simulink model "dbt_ut"  (Simulink 8.1)
settings: Solver=FixedStepDiscrete  StartTime=0.0  StopTime=Inf  FixedStep=0.005  RelTol=1e-3
PostLoadFcn:
  | , if any(exist('dsrtsu_mdlpostloadfcn', 'file') == [2, 3, 6]), try dsrtsu_mdlpostloadfcn('Execute', bdroot); catch fprintf('Error in PostLoadFcn (dsrtsu_mdlpostloadfcn) for model "%s":\n %s\n', bdroot, lasterr); end, end,
libraries: siltestlib x6, dbt x1
settings Model: DSRTSU_INTERNAL_RTI_VER=450  DSRTSU_INTERNAL_RTI_TYPE=rti1401  RTICANMMDATA=struct('GeneralSetupData',struct('modelroot','D:\ELN150201_TAIWAN\trunk\AdasDragon\software\sw_development\arch\app\acc','generalsettings',struct('filesettings',struct('destfolder',struct('Name','RTICANMM_FILES','Check',1),'buildfolder',struct('Name','.','Check',1),'AbsDestfolder',struct('Name','D:\ELN150201_TAIWAN\trunk\AdasDragon\software\sw_development\arch\app\acc\RTICANMM_FILES'),'AbsBuildfolder',struct('Name','D:\ELN150201_TAIWAN\trunk\AdasDragon\software\sw_development\arch\app\acc'))),'options',struct('addpaths',1,'rmpaths',1,'addtrcexclusion',logical(1),'cannavigator',struct('checkmonitoring',0),'show_usrtrc',0,'use_usrtrc',0),'advanced',struct('options',[1 1 1 1 1 1 1 1 1 1 1 1 1 1 1 1 1 1 1 1 1 1 1 1 1 1 1 1 1 1 1 1 1 1 1 1 1 1 1 1 1 1 1 1 1 1 1 1 1 1 1 1 1 1 1 1 1 1 1 1 1 1 1 1 1 1 1 1 1 1 1 1 1 1 1 1 1 1 1 1 1 1 1 1 1 1 1 1 1 1 1 1 1 1 1 1 1 1 1 1]),'MPSetup',{{}},'modelname','dbt_ut','block','dbt_ut'))  DSRTSU_INTERNAL_RTIFPGA=40  Creator=AT015555  LastModifiedBy=AT015555  BufferReuse=off
settings DataIOCC: SignalLoggingSaveFormat=Dataset
settings OptimizationCC: BlockReduction=off  OptimizeBlockIOStorage=off  BufferReuse=off  ExpressionFolding=off  ExpressionDepthLimit=128  LocalBlockOutputs=off
settings DebuggingCC: FcnCallInpInsideContextMsg=EnableAllAsError
settings HardwareCC: ProdIntDivRoundTo=Zero  ProdEndianess=BigEndian  ProdHWDeviceType=Generic->Custom  TargetIntDivRoundTo=Zero  TargetEndianess=BigEndian  TargetHWDeviceType=Generic->Custom
settings RTWCC: SystemTargetFile=rti1401.tlc  MakeCommand=make_rti  TemplateMakefile=rti1401.tmf  Description=dSPACE DS1401 Hardware Platform  ProcessScript=rti1401_make_rtw_hook
settings STFCustomTargetCC: CodeReplacementLibrary=ANSI_C  ParMdlRefBuildCompliant=on  GeneratePreprocessorConditionals=Disable all  MatFileLogging=on  SystemTargetFile=rti1401.tlc
settings GRTTargetCC: CompOptLevelCompliant=off  ConcurrentExecutionCompliant=off  ExtModeMexFile=noextcomm
settings CustomProperty: DataType=RTWOptions_EnumType_C__Program Files (x86)_dSPACE RCPHIL 2014-B_MATLAB_RTI_RTI1401_TLC_rti1401_1InitialSimState  Value=RUN
settings EnumStrPairs: String=RUN

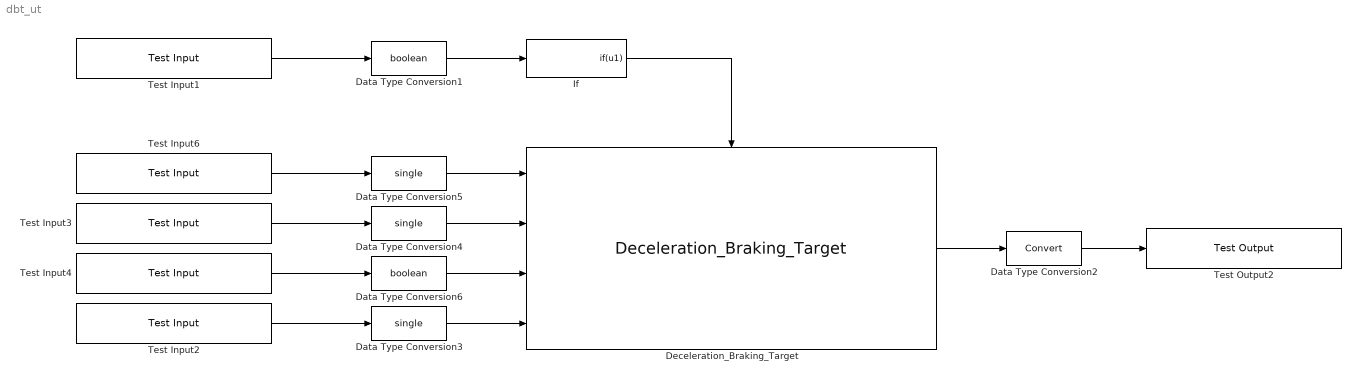
== system dbt_ut ==
  Data Type Conversion1 : DataTypeConversion  OutDataTypeStr=boolean
  Data Type Conversion2 : DataTypeConversion
  Data Type Conversion3 : DataTypeConversion  OutDataTypeStr=single
  Data Type Conversion4 : DataTypeConversion  OutDataTypeStr=single
  Data Type Conversion5 : DataTypeConversion  OutDataTypeStr=single
  Data Type Conversion6 : DataTypeConversion  OutDataTypeStr=boolean
  Deceleration_Braking_Target : dbt/Deceleration_Braking_Target
  If : If  IfExpression=u1  ShowElse=off
  Test Input1 : siltestlib/Test Input  varname=Block_Enable  sampletime=0.005
  Test Input2 : siltestlib/Test Input  varname=VIFO_ACCTargetVehRelSpeedX_mps  sampletime=0.005
  Test Input3 : siltestlib/Test Input  varname=VJUD_ACCSetTimeGap_s  sampletime=0.005
  Test Input4 : siltestlib/Test Input  varname=VACC_ACCBrakeReleaseSituation_flg  sampletime=0.005
  Test Input6 : siltestlib/Test Input  varname=VACC_ACCMCDecel_mps2  sampletime=0.005
  Test Output2 : siltestlib/Test Output  varname=VACC_ACCDecelTargetBraking_mps2  sampletime=-1
  wires:
  Test Input6/1 -> Data Type Conversion5/1
  Data Type Conversion5/1 -> Deceleration_Braking_Target/1
  Test Input1/1 -> Data Type Conversion1/1
  Data Type Conversion2/1 -> Test Output2/1
  Deceleration_Braking_Target/1 -> Data Type Conversion2/1
  Test Input2/1 -> Data Type Conversion3/1
  Data Type Conversion3/1 -> Deceleration_Braking_Target/4
  Test Input3/1 -> Data Type Conversion4/1
  Data Type Conversion4/1 -> Deceleration_Braking_Target/2
  Test Input4/1 -> Data Type Conversion6/1
  Data Type Conversion6/1 -> Deceleration_Braking_Target/3
  Data Type Conversion1/1 -> If/1
  If/1 -> Deceleration_Braking_Target/Action
